simulink model "c00003"  (R2018a)
settings: Solver=ode3  StartTime=0.0  StopTime=10.0  RelTol=1e-3  EnableMultiTasking=on
undefined symbols (not defined in the file): b, DiscIntNeverNeededParam, J, K, L, PosMinimaW3, PosMinimaW4, R
settings Model: Creator=aarrieta  LastModifiedBy=umarkiegi
settings DataIOCC: LimitDataPoints=on  SaveFormat=Array
settings OptimizationCC: LifeSpan=inf
settings DebuggingCC: UnderspecifiedInitializationDetection=Classic  MergeDetectMultiDrivingBlocksExec=none  SolverPrmCheckMsg=warning  StateNameClashWarn=warning  SFUnexpectedBacktrackingDiag=warning  SFNoUnconditionalDefaultTransitionDiag=warning  SFExecutionAtInitializationDiag=none
settings HardwareCC: ProdBitPerPointer=32  ProdBitPerSizeT=32  ProdBitPerPtrDiffT=32  ProdLargestAtomicFloat=None  ProdIntDivRoundTo=Undefined  ProdEndianess=Unspecified  ProdWordSize=32  ProdHWDeviceType=32-bit Generic
settings ModelReferenceCC: PropagateSignalLabelsOutOfModel=off
settings CodeAppCC: StateflowObjectComments=on
settings GRTTargetCC: TargetLangStandard=C89/C90 (ANSI)  GeneratePreprocessorConditionals=Disable all
settings ConfigComp: CovMetricSettings=dw  CovHtmlReporting=on  CovSaveCumulativeToWorkspaceVar=on  CovSaveSingleToWorkspaceVar=on  CovExternalEMLEnable=off  DVMaxTestCaseSteps=20  DVTestSuiteOptimization=CombinedObjectives (Nonlinear Extended)  DVDetectFloatOverflow=off

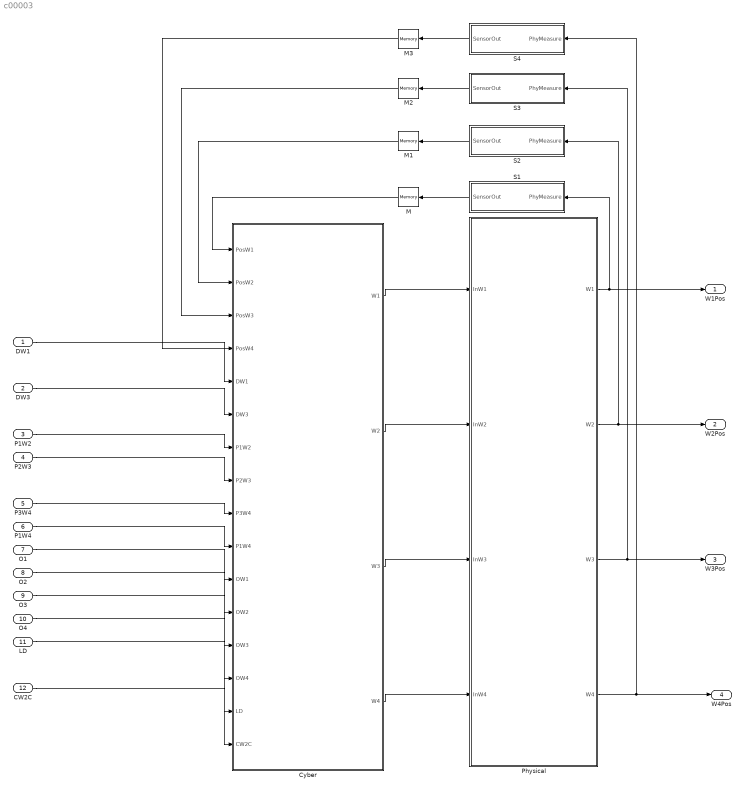
== system c00003 ==
  DW1 : Inport  OutMin=0  OutMax=4  OutDataTypeStr=int8
  DW3 : Inport  Port=2  OutMin=0  OutMax=4  OutDataTypeStr=int8
  P1W2 : Inport  Port=3  OutMin=0  OutMax=4  OutDataTypeStr=int8
  P2W3 : Inport  Port=4  OutMin=0  OutMax=4  OutDataTypeStr=int8
  P3W4 : Inport  Port=5  OutMin=0  OutMax=4  OutDataTypeStr=int8
  P1W4 : Inport  Port=6  OutMin=0  OutMax=4  OutDataTypeStr=int8
  O1 : Inport  Port=7  OutDataTypeStr=boolean
  O2 : Inport  Port=8  OutDataTypeStr=boolean
  O3 : Inport  Port=9  OutDataTypeStr=boolean
  O4 : Inport  Port=10  OutDataTypeStr=boolean
  LD : Inport  Port=11  OutDataTypeStr=boolean
  CW2C : Inport  Port=12  OutMin=0  OutMax=4  OutDataTypeStr=int8
  Cyber : Subsystem
  M{,1..3} (4 alike) : Memory
  Physical : Subsystem
  S1 : Subsystem
  S2 : Subsystem
  S3 : Subsystem
  S4 : Subsystem
  W1Pos : Outport
  W2Pos : Outport  Port=2
  W3Pos : Outport  Port=3
  W4Pos : Outport  Port=4
  wires:
  Cyber/3(W3) -> Physical/3(InW3)
  Physical/1(W1) -> W1Pos/1, S1/1(PhyMeasure)
  Physical/2(W2) -> W2Pos/1, S2/1(PhyMeasure)
  Physical/3(W3) -> W3Pos/1, S3/1(PhyMeasure)
  Physical/4(W4) -> W4Pos/1, S4/1(PhyMeasure)
  M/1 -> Cyber/1(PosW1)
  M1/1 -> Cyber/2(PosW2)
  Cyber/4(W4) -> Physical/4(InW4)
  Cyber/2(W2) -> Physical/2(InW2)
  Cyber/1(W1) -> Physical/1(InW1)
  S4/1(SensorOut) -> M3/1
  M2/1 -> Cyber/3(PosW3)
  S3/1(SensorOut) -> M2/1
  S2/1(SensorOut) -> M1/1
  S1/1(SensorOut) -> M/1
  DW1/1 -> Cyber/5(DW1)
  DW3/1 -> Cyber/6(DW3)
  P1W2/1 -> Cyber/7(P1W2)
  P2W3/1 -> Cyber/8(P2W3)
  P3W4/1 -> Cyber/9(P3W4)
  P1W4/1 -> Cyber/10(P1W4)
  O1/1 -> Cyber/11(OW1)
  O2/1 -> Cyber/12(OW2)
  O3/1 -> Cyber/13(OW3)
  O4/1 -> Cyber/14(OW4)
  LD/1 -> Cyber/15(LD)
  CW2C/1 -> Cyber/16(CW2C)
  M3/1 -> Cyber/4(PosW4)

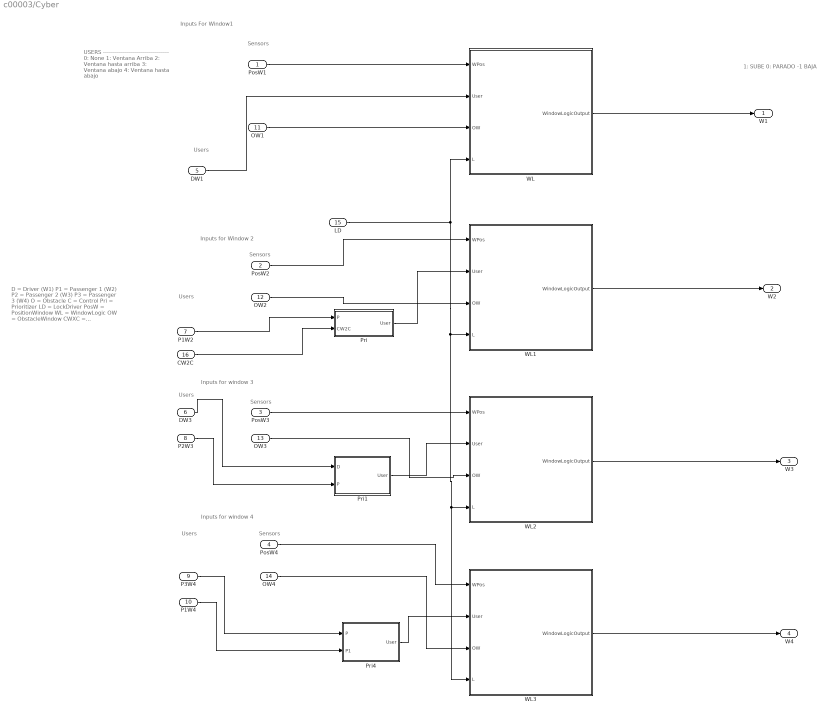
== system c00003/Cyber ==
  note: D = Driver (W1)
      | P1 = Passenger 1 (W2)
      | P2 = Passenger 2 (W3)
      | P3 = Passenger 3 (W4)
      | O = Obstacle
      | C = Control
      | Pri = Prioritizer
      | LD = LockDriver
      | PosW = PositionWindow
      | WL = WindowLogic
      | OW = ObstacleWindow
      | CWXC = ControlWindowXCentralized
      | S = Sensor
      | L = Lock
      | WPos = WindowPosition
      | M = Memory
      | InW = InputWindow
      | WIn = WindowInput
  note: 1: SUBE
      | 0: PARADO
      | -1 BAJA
  note: USERS
      | ---------------------------------
      | 0: None
      | 1: Ventana Arriba
      | 2: Ventana hasta arriba
      | 3: Ventana abajo
      | 4: Ventana hasta abajo
  note: Sensors
  note: Users
  note: Sensors
  note: Users
  note: Sensors
  note: Users
  note: Users
  note: Inputs for window 4
  note: Inputs for window 3
  note: Inputs for Window 2
  note: Inputs For Window1
  note: Sensors
  PosW1 : Inport
  PosW2 : Inport  Port=2
  PosW3 : Inport  Port=3
  PosW4 : Inport  Port=4
  DW1 : Inport  Port=5
  DW3 : Inport  Port=6
  P1W2 : Inport  Port=7
  P2W3 : Inport  Port=8
  P3W4 : Inport  Port=9
  P1W4 : Inport  Port=10
  OW1 : Inport  Port=11
  OW2 : Inport  Port=12
  OW3 : Inport  Port=13
  OW4 : Inport  Port=14
  LD : Inport  Port=15
  CW2C : Inport  Port=16
  Pri : Subsystem
  Pri1 : Subsystem
  Pri4 : Subsystem
  WL : Subsystem
  WL1 : Subsystem
  WL2 : Subsystem
  WL3 : Subsystem
  W1 : Outport
  W2 : Outport  Port=2
  W3 : Outport  Port=3
  W4 : Outport  Port=4
  wires:
  LD/1 -> WL/4(L), WL1/4(L), WL3/4(L), WL2/4(L)
  PosW1/1 -> WL/1(WPos)
  OW1/1 -> WL/3(OW)
  WL/1(WindowLogicOutput) -> W1/1
  Pri/1(User) -> WL1/2(User)
  P1W2/1 -> Pri/1(P)
  PosW2/1 -> WL1/1(WPos)
  OW2/1 -> WL1/3(OW)
  WL1/1(WindowLogicOutput) -> W2/1
  Pri1/1(User) -> WL2/2(User)
  PosW3/1 -> WL2/1(WPos)
  OW3/1 -> WL2/3(OW)
  DW3/1 -> Pri1/1(D)
  P2W3/1 -> Pri1/2(P)
  P3W4/1 -> Pri4/1(P)
  P1W4/1 -> Pri4/2(P1)
  PosW4/1 -> WL3/1(WPos)
  OW4/1 -> WL3/3(OW)
  Pri4/1(User) -> WL3/2(User)
  WL2/1(WindowLogicOutput) -> W3/1
  WL3/1(WindowLogicOutput) -> W4/1
  CW2C/1 -> Pri/2(CW2C)
  DW1/1 -> WL/2(User)

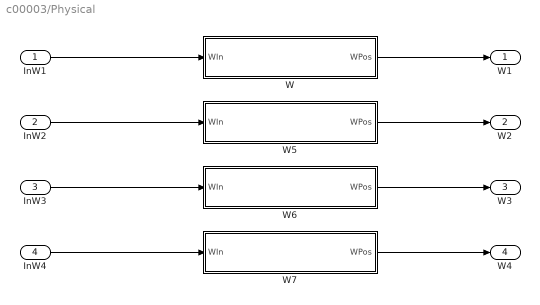
== system c00003/Physical ==
  InW1 : Inport
  InW2 : Inport  Port=2
  InW3 : Inport  Port=3
  InW4 : Inport  Port=4
  W : Subsystem
  W5 : Subsystem
  W6 : Subsystem
  W7 : Subsystem
  W1 : Outport
  W2 : Outport  Port=2
  W3 : Outport  Port=3
  W4 : Outport  Port=4
  wires:
  InW1/1 -> W/1(WIn)
  InW2/1 -> W5/1(WIn)
  InW3/1 -> W6/1(WIn)
  InW4/1 -> W7/1(WIn)
  W/1(WPos) -> W1/1
  W5/1(WPos) -> W2/1
  W6/1(WPos) -> W3/1
  W7/1(WPos) -> W4/1

== system c00003/S1 ==
  PhyMeasure : Inport
  SensorOut : Outport
  wires:
  PhyMeasure/1 -> SensorOut/1

== system c00003/S2 ==
  PhyMeasure : Inport
  SensorOut : Outport
  wires:
  PhyMeasure/1 -> SensorOut/1

== system c00003/S3 ==
  PhyMeasure : Inport
  SensorOut : Outport
  wires:
  PhyMeasure/1 -> SensorOut/1

== system c00003/S4 ==
  PhyMeasure : Inport
  SensorOut : Outport
  wires:
  PhyMeasure/1 -> SensorOut/1

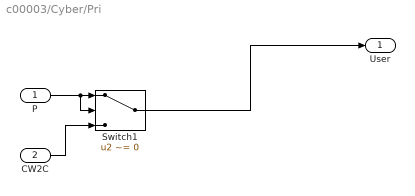
== system c00003/Cyber/Pri ==
  P : Inport
  CW2C : Inport  Port=2
  Switch1 : Switch  Criteria=u2 ~= 0
  User : Outport
  wires:
  P/1 -> Switch1/2, Switch1/1
  CW2C/1 -> Switch1/3
  Switch1/1 -> User/1

== system c00003/Cyber/Pri1 ==
  D : Inport
  P : Inport  Port=2
  Switch : Switch  Criteria=u2 ~= 0
  User : Outport
  wires:
  Switch/1 -> User/1
  D/1 -> Switch/1, Switch/2
  P/1 -> Switch/3

== system c00003/Cyber/Pri4 ==
  P : Inport
  P1 : Inport  Port=2
  Switch1 : Switch  Criteria=u2 ~= 0
  User : Outport
  wires:
  P/1 -> Switch1/2, Switch1/1
  P1/1 -> Switch1/3
  Switch1/1 -> User/1

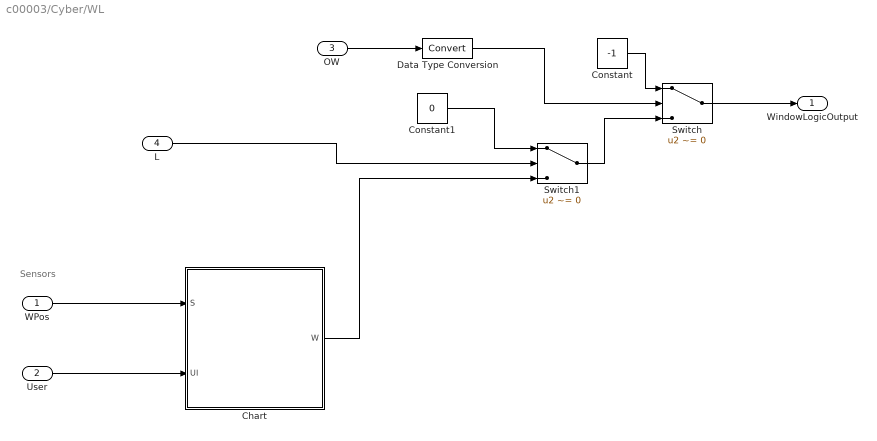
== system c00003/Cyber/WL ==
  note: Sensors
  WPos : Inport
  User : Inport  Port=2
  OW : Inport  Port=3
  L : Inport  Port=4
  Chart : Stateflow chart  TreatAsAtomicUnit=on
  Constant : Constant  Value=-1
  Constant1 : Constant  Value=0
  Data Type Conversion : DataTypeConversion
  Switch : Switch  Criteria=u2 ~= 0  Threshold=1  ZeroCross=off
  Switch1 : Switch  Criteria=u2 ~= 0
  WindowLogicOutput : Outport
  wires:
  OW/1 -> Data Type Conversion/1
  Switch/1 -> WindowLogicOutput/1
  Constant1/1 -> Switch1/1
  Switch1/1 -> Switch/3
  WPos/1 -> Chart/1(S)
  User/1 -> Chart/2(UI)
  Chart/1(W) -> Switch1/3
  Constant/1 -> Switch/1
  Data Type Conversion/1 -> Switch/2
  L/1 -> Switch1/2

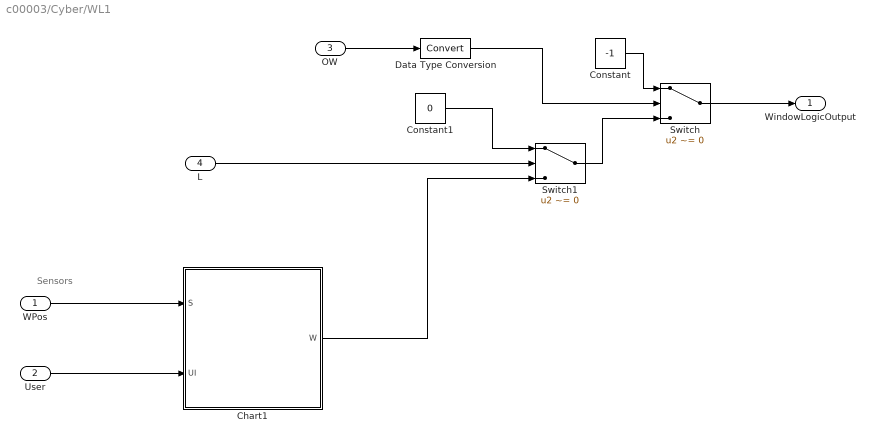
== system c00003/Cyber/WL1 ==
  note: Sensors
  WPos : Inport
  User : Inport  Port=2
  OW : Inport  Port=3
  L : Inport  Port=4
  Chart1 : Stateflow chart  TreatAsAtomicUnit=on
  Constant : Constant  Value=-1
  Constant1 : Constant  Value=0
  Data Type Conversion : DataTypeConversion
  Switch : Switch  Criteria=u2 ~= 0  Threshold=1  ZeroCross=off
  Switch1 : Switch  Criteria=u2 ~= 0
  WindowLogicOutput : Outport
  wires:
  L/1 -> Switch1/2
  Data Type Conversion/1 -> Switch/2
  Constant/1 -> Switch/1
  Chart1/1(W) -> Switch1/3
  User/1 -> Chart1/2(UI)
  WPos/1 -> Chart1/1(S)
  Switch1/1 -> Switch/3
  Constant1/1 -> Switch1/1
  Switch/1 -> WindowLogicOutput/1
  OW/1 -> Data Type Conversion/1

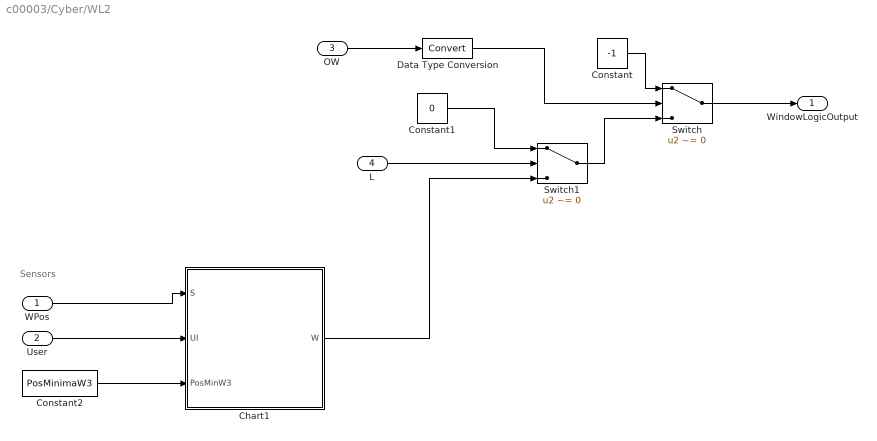
== system c00003/Cyber/WL2 ==
  note: Sensors
  WPos : Inport
  User : Inport  Port=2
  OW : Inport  Port=3
  L : Inport  Port=4
  Chart1 : Stateflow chart  TreatAsAtomicUnit=on
  Constant : Constant  Value=-1
  Constant1 : Constant  Value=0
  Constant2 : Constant  Value=PosMinimaW3
  Data Type Conversion : DataTypeConversion
  Switch : Switch  Criteria=u2 ~= 0  Threshold=1  ZeroCross=off
  Switch1 : Switch  Criteria=u2 ~= 0
  WindowLogicOutput : Outport
  wires:
  OW/1 -> Data Type Conversion/1
  Switch/1 -> WindowLogicOutput/1
  Constant1/1 -> Switch1/1
  Switch1/1 -> Switch/3
  WPos/1 -> Chart1/1(S)
  User/1 -> Chart1/2(UI)
  Chart1/1(W) -> Switch1/3
  Constant/1 -> Switch/1
  Data Type Conversion/1 -> Switch/2
  L/1 -> Switch1/2
  Constant2/1 -> Chart1/3(PosMinW3)

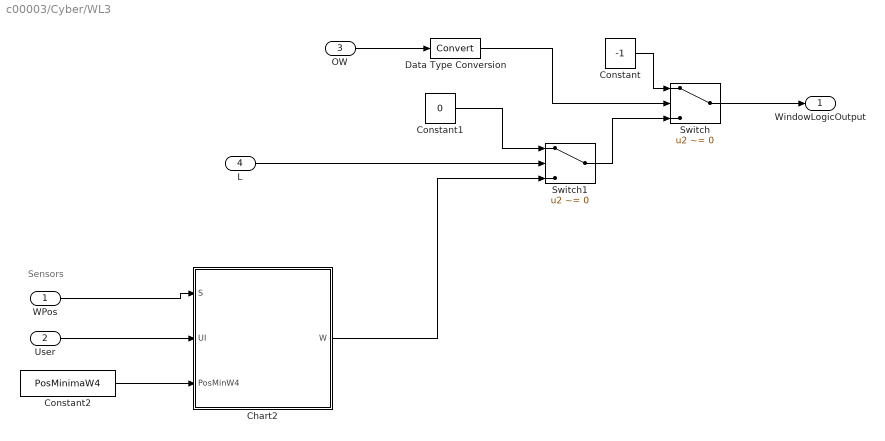
== system c00003/Cyber/WL3 ==
  note: Sensors
  WPos : Inport
  User : Inport  Port=2
  OW : Inport  Port=3
  L : Inport  Port=4
  Chart2 : Stateflow chart  TreatAsAtomicUnit=on
  Constant : Constant  Value=-1
  Constant1 : Constant  Value=0
  Constant2 : Constant  Value=PosMinimaW4
  Data Type Conversion : DataTypeConversion
  Switch : Switch  Criteria=u2 ~= 0  Threshold=1  ZeroCross=off
  Switch1 : Switch  Criteria=u2 ~= 0
  WindowLogicOutput : Outport
  wires:
  L/1 -> Switch1/2
  Data Type Conversion/1 -> Switch/2
  Constant/1 -> Switch/1
  Chart2/1(W) -> Switch1/3
  User/1 -> Chart2/2(UI)
  WPos/1 -> Chart2/1(S)
  Switch1/1 -> Switch/3
  Constant1/1 -> Switch1/1
  Switch/1 -> WindowLogicOutput/1
  OW/1 -> Data Type Conversion/1
  Constant2/1 -> Chart2/3(PosMinW4)

== system c00003/Physical/W ==
  WIn : Inport
  DC_Engine : Subsystem
  Discrete-Time Integrator : DiscreteIntegrator  InitialCondition=5  SampleTime=-1  LimitOutput=on  UpperSaturationLimit=5  LowerSaturationLimit=0  ICPrevOutput=DiscIntNeverNeededParam  ICPrevScaledInput=DiscIntNeverNeededParam
  WPos : Outport
  wires:
  Discrete-Time Integrator/1 -> WPos/1
  DC_Engine/1(Speed) -> Discrete-Time Integrator/1
  WIn/1 -> DC_Engine/1(input)

== system c00003/Physical/W5 ==
  WIn : Inport
  DC_Engine : Subsystem
  Discrete-Time Integrator : DiscreteIntegrator  InitialCondition=5  SampleTime=-1  LimitOutput=on  UpperSaturationLimit=5  LowerSaturationLimit=0  ICPrevOutput=DiscIntNeverNeededParam  ICPrevScaledInput=DiscIntNeverNeededParam
  WPos : Outport
  wires:
  WIn/1 -> DC_Engine/1(input)
  DC_Engine/1(Speed) -> Discrete-Time Integrator/1
  Discrete-Time Integrator/1 -> WPos/1

== system c00003/Physical/W6 ==
  WIn : Inport
  DC_Engine : Subsystem
  Discrete-Time Integrator : DiscreteIntegrator  InitialCondition=5  SampleTime=-1  LimitOutput=on  UpperSaturationLimit=5  LowerSaturationLimit=PosMinimaW3  ICPrevOutput=DiscIntNeverNeededParam  ICPrevScaledInput=DiscIntNeverNeededParam
  WPos : Outport
  wires:
  Discrete-Time Integrator/1 -> WPos/1
  DC_Engine/1(Speed) -> Discrete-Time Integrator/1
  WIn/1 -> DC_Engine/1(input)

== system c00003/Physical/W7 ==
  WIn : Inport
  DC_Engine : Subsystem
  Discrete-Time Integrator : DiscreteIntegrator  InitialCondition=5  SampleTime=-1  LimitOutput=on  UpperSaturationLimit=5  LowerSaturationLimit=PosMinimaW4  ICPrevOutput=DiscIntNeverNeededParam  ICPrevScaledInput=DiscIntNeverNeededParam
  WPos : Outport
  wires:
  WIn/1 -> DC_Engine/1(input)
  DC_Engine/1(Speed) -> Discrete-Time Integrator/1
  Discrete-Time Integrator/1 -> WPos/1

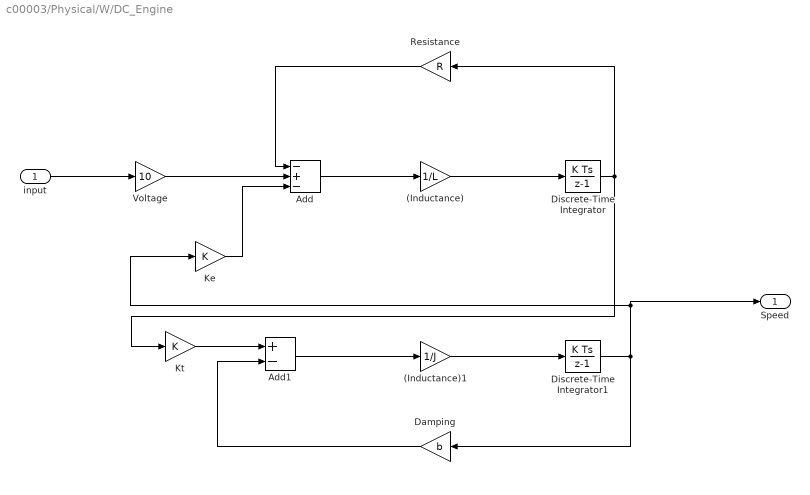
== system c00003/Physical/W/DC_Engine ==
  input : Inport
  (Inductance) : Gain  Gain=1/L
  (Inductance)1 : Gain  Gain=1/J
  Add : Sum  Inputs=-+-
  Add1 : Sum  Inputs=+-
  Damping : Gain  Gain=b
  Discrete-Time Integrator : DiscreteIntegrator  SampleTime=-1  ICPrevOutput=DiscIntNeverNeededParam  ICPrevScaledInput=DiscIntNeverNeededParam
  Discrete-Time Integrator1 : DiscreteIntegrator  SampleTime=-1  ICPrevOutput=DiscIntNeverNeededParam  ICPrevScaledInput=DiscIntNeverNeededParam
  Ke : Gain  Gain=K
  Kt : Gain  Gain=K
  Resistance : Gain  Gain=R
  Voltage : Gain  Gain=10
  Speed : Outport
  wires:
  input/1 -> Voltage/1
  Voltage/1 -> Add/2
  Add/1 -> (Inductance)/1
  Discrete-Time Integrator/1 -> Kt/1, Resistance/1
  Resistance/1 -> Add/1
  Ke/1 -> Add/3
  Kt/1 -> Add1/1
  Add1/1 -> (Inductance)1/1
  (Inductance)1/1 -> Discrete-Time Integrator1/1
  Discrete-Time Integrator1/1 -> Ke/1, Speed/1, Damping/1
  Damping/1 -> Add1/2
  (Inductance)/1 -> Discrete-Time Integrator/1

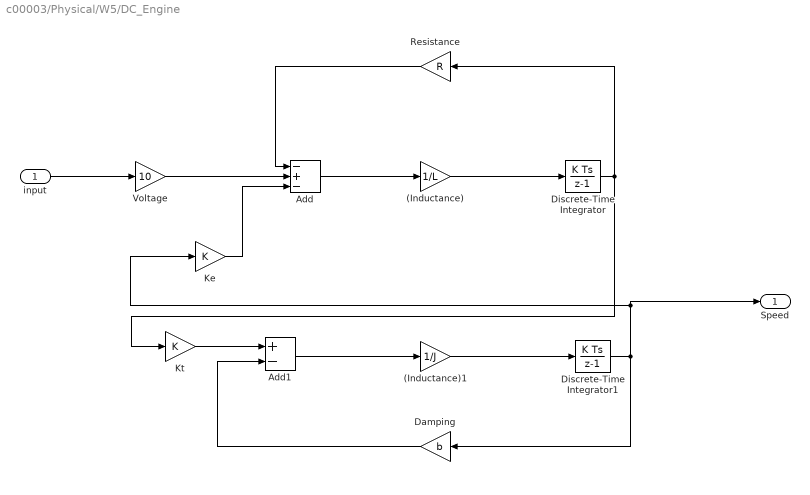
== system c00003/Physical/W5/DC_Engine ==
  input : Inport
  (Inductance) : Gain  Gain=1/L
  (Inductance)1 : Gain  Gain=1/J
  Add : Sum  Inputs=-+-
  Add1 : Sum  Inputs=+-
  Damping : Gain  Gain=b
  Discrete-Time Integrator : DiscreteIntegrator  SampleTime=-1  ICPrevOutput=DiscIntNeverNeededParam  ICPrevScaledInput=DiscIntNeverNeededParam
  Discrete-Time Integrator1 : DiscreteIntegrator  SampleTime=-1  ICPrevOutput=DiscIntNeverNeededParam  ICPrevScaledInput=DiscIntNeverNeededParam
  Ke : Gain  Gain=K
  Kt : Gain  Gain=K
  Resistance : Gain  Gain=R
  Voltage : Gain  Gain=10
  Speed : Outport
  wires:
  Damping/1 -> Add1/2
  Discrete-Time Integrator1/1 -> Damping/1, Speed/1, Ke/1
  (Inductance)1/1 -> Discrete-Time Integrator1/1
  Add1/1 -> (Inductance)1/1
  Kt/1 -> Add1/1
  Ke/1 -> Add/3
  Resistance/1 -> Add/1
  Discrete-Time Integrator/1 -> Resistance/1, Kt/1
  (Inductance)/1 -> Discrete-Time Integrator/1
  Add/1 -> (Inductance)/1
  Voltage/1 -> Add/2
  input/1 -> Voltage/1

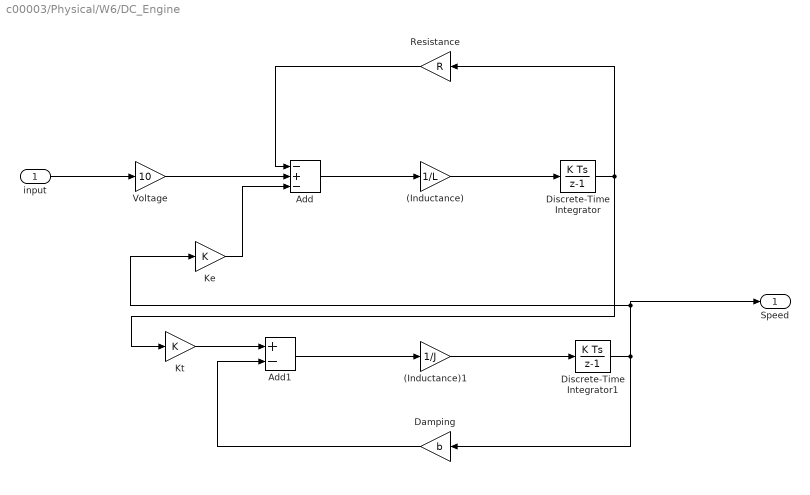
== system c00003/Physical/W6/DC_Engine ==
  input : Inport
  (Inductance) : Gain  Gain=1/L
  (Inductance)1 : Gain  Gain=1/J
  Add : Sum  Inputs=-+-
  Add1 : Sum  Inputs=+-
  Damping : Gain  Gain=b
  Discrete-Time Integrator : DiscreteIntegrator  SampleTime=-1  ICPrevOutput=DiscIntNeverNeededParam  ICPrevScaledInput=DiscIntNeverNeededParam
  Discrete-Time Integrator1 : DiscreteIntegrator  SampleTime=-1  ICPrevOutput=DiscIntNeverNeededParam  ICPrevScaledInput=DiscIntNeverNeededParam
  Ke : Gain  Gain=K
  Kt : Gain  Gain=K
  Resistance : Gain  Gain=R
  Voltage : Gain  Gain=10
  Speed : Outport
  wires:
  input/1 -> Voltage/1
  Voltage/1 -> Add/2
  Add/1 -> (Inductance)/1
  (Inductance)/1 -> Discrete-Time Integrator/1
  Discrete-Time Integrator/1 -> Kt/1, Resistance/1
  Resistance/1 -> Add/1
  Ke/1 -> Add/3
  Kt/1 -> Add1/1
  Add1/1 -> (Inductance)1/1
  (Inductance)1/1 -> Discrete-Time Integrator1/1
  Discrete-Time Integrator1/1 -> Ke/1, Speed/1, Damping/1
  Damping/1 -> Add1/2

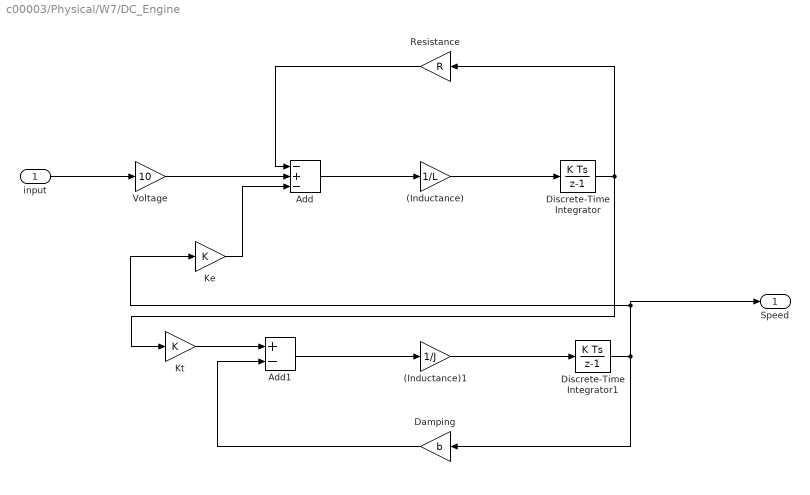
== system c00003/Physical/W7/DC_Engine ==
  input : Inport
  (Inductance) : Gain  Gain=1/L
  (Inductance)1 : Gain  Gain=1/J
  Add : Sum  Inputs=-+-
  Add1 : Sum  Inputs=+-
  Damping : Gain  Gain=b
  Discrete-Time Integrator : DiscreteIntegrator  SampleTime=-1  ICPrevOutput=DiscIntNeverNeededParam  ICPrevScaledInput=DiscIntNeverNeededParam
  Discrete-Time Integrator1 : DiscreteIntegrator  SampleTime=-1  ICPrevOutput=DiscIntNeverNeededParam  ICPrevScaledInput=DiscIntNeverNeededParam
  Ke : Gain  Gain=K
  Kt : Gain  Gain=K
  Resistance : Gain  Gain=R
  Voltage : Gain  Gain=10
  Speed : Outport
  wires:
  Damping/1 -> Add1/2
  Discrete-Time Integrator1/1 -> Damping/1, Speed/1, Ke/1
  (Inductance)1/1 -> Discrete-Time Integrator1/1
  Add1/1 -> (Inductance)1/1
  Kt/1 -> Add1/1
  Ke/1 -> Add/3
  Resistance/1 -> Add/1
  Discrete-Time Integrator/1 -> Resistance/1, Kt/1
  (Inductance)/1 -> Discrete-Time Integrator/1
  Add/1 -> (Inductance)/1
  Voltage/1 -> Add/2
  input/1 -> Voltage/1

== stateflow chart c00003/Cyber/WL/Chart ==
  state Bajand_hasta_abajo
    entry: W = -1;
  state Bajando
    entry: W = -1;
  state Idle
    entry:W = 0;
  state Subiendo_hasta_arriba
    entry: W = 1;
  state Subiendo
    entry: W = 1;
  Subiendo -> Bajand_hasta_abajo [order 4] : [UI==4]
  Bajand_hasta_abajo -> Bajando [order 2] : [UI==3]
  Subiendo -> Bajando [order 3] : [UI==3]
  Bajando -> Bajand_hasta_abajo [order 2] : [UI==4]
  Idle -> Bajando [order 3] : [UI==3&&S>0]
  Subiendo_hasta_arriba -> Bajand_hasta_abajo [order 3] : [UI==4]
  Idle -> Bajand_hasta_abajo [order 4] : [UI==4&&S>0]
  Bajando -> Subiendo [order 3] : [UI==1]
  Subiendo_hasta_arriba -> Bajando [order 4] : [UI==3]
  Bajand_hasta_abajo -> Subiendo [order 4] : [UI==1]
  Bajand_hasta_abajo -> Idle [order 1] : [S<=0]
  Bajand_hasta_abajo -> Subiendo_hasta_arriba [order 3] : [UI==2]
  Bajando -> Idle [order 1] : [S<=0||UI==0]
  Bajando -> Subiendo_hasta_arriba [order 4] : [UI==2]
  (default) -> Idle
  Idle -> Subiendo_hasta_arriba [order 2] : [UI==2&&S<5]
  Idle -> Subiendo [order 1] : [UI == 1&&S<5]
  Subiendo -> Idle [order 1] : [S>=5||UI==0]
  Subiendo_hasta_arriba -> Idle [order 1] : [S >=5]
  Subiendo_hasta_arriba -> Subiendo [order 2] : [UI ==1]
  Subiendo -> Subiendo_hasta_arriba [order 2] : [UI==2]
  data: S input; UI input; W output double

== stateflow chart c00003/Cyber/WL2/Chart1 ==
  state Bajand_hasta_abajo
    entry: W = -1;
  state Bajando
    entry: W = -1;
  state Idle
    entry:W = 0;
  state Subiendo_hasta_arriba
    entry: W = 1;
  state Subiendo
    entry: W = 1;
  Subiendo -> Bajand_hasta_abajo [order 4] : [UI==4]
  Bajand_hasta_abajo -> Bajando [order 2] : [UI==3]
  Subiendo -> Bajando [order 3] : [UI==3]
  Bajando -> Bajand_hasta_abajo [order 2] : [UI==4]
  Idle -> Bajando [order 3] : [UI==3&&S>PosMinW3]
  Subiendo_hasta_arriba -> Bajand_hasta_abajo [order 3] : [UI==4]
  Idle -> Bajand_hasta_abajo [order 4] : [UI==4&&S>PosMinW3]
  Bajando -> Subiendo [order 3] : [UI==1]
  Subiendo_hasta_arriba -> Bajando [order 4] : [UI==3]
  Bajand_hasta_abajo -> Subiendo [order 4] : [UI==1]
  Bajand_hasta_abajo -> Idle [order 1] : [S<=PosMinW3]
  Bajand_hasta_abajo -> Subiendo_hasta_arriba [order 3] : [UI==2]
  Bajando -> Idle [order 1] : [S<=PosMinW3||UI==0]
  Bajando -> Subiendo_hasta_arriba [order 4] : [UI==2]
  (default) -> Idle
  Idle -> Subiendo_hasta_arriba [order 2] : [UI==2&&S<5]
  Idle -> Subiendo [order 1] : [UI == 1&&S<5]
  Subiendo -> Idle [order 1] : [S>=5||UI==0]
  Subiendo_hasta_arriba -> Idle [order 1] : [S >=5]
  Subiendo_hasta_arriba -> Subiendo [order 2] : [UI ==1]
  Subiendo -> Subiendo_hasta_arriba [order 2] : [UI==2]
  data: S input; UI input; W output double; PosMinW3 input

== stateflow chart c00003/Cyber/WL1/Chart1 ==
  state Bajand_hasta_abajo
    entry: W = -1;
  state Bajando
    entry: W = -1;
  state Idle
    entry:W = 0;
  state Subiendo_hasta_arriba
    entry: W = 1;
  state Subiendo
    entry: W = 1;
  Subiendo -> Bajand_hasta_abajo [order 4] : [UI==4]
  Bajand_hasta_abajo -> Bajando [order 2] : [UI==3]
  Subiendo -> Bajando [order 3] : [UI==3]
  Bajando -> Bajand_hasta_abajo [order 2] : [UI==4]
  Idle -> Bajando [order 3] : [UI==3&&S>0]
  Subiendo_hasta_arriba -> Bajand_hasta_abajo [order 3] : [UI==4]
  Idle -> Bajand_hasta_abajo [order 4] : [UI==4&&S>0]
  Bajando -> Subiendo [order 3] : [UI==1]
  Subiendo_hasta_arriba -> Bajando [order 4] : [UI==3]
  Bajand_hasta_abajo -> Subiendo [order 4] : [UI==1]
  Bajand_hasta_abajo -> Idle [order 1] : [S<=0]
  Bajand_hasta_abajo -> Subiendo_hasta_arriba [order 3] : [UI==2]
  Bajando -> Idle [order 1] : [S<=0||UI==0]
  Bajando -> Subiendo_hasta_arriba [order 4] : [UI==2]
  (default) -> Idle
  Idle -> Subiendo_hasta_arriba [order 2] : [UI==2&&S<5]
  Idle -> Subiendo [order 1] : [UI == 1&&S<5]
  Subiendo -> Idle [order 1] : [S>=5||UI==0]
  Subiendo_hasta_arriba -> Idle [order 1] : [S >=5]
  Subiendo_hasta_arriba -> Subiendo [order 2] : [UI ==1]
  Subiendo -> Subiendo_hasta_arriba [order 2] : [UI==2]
  data: S input; UI input; W output double

== stateflow chart c00003/Cyber/WL3/Chart2 ==
  state Bajand_hasta_abajo
    entry: W = -1;
  state Bajando
    entry: W = -1;
  state Idle
    entry:W = 0;
  state Subiendo_hasta_arriba
    entry: W = 1;
  state Subiendo
    entry: W = 1;
  Subiendo -> Bajand_hasta_abajo [order 4] : [UI==4]
  Bajand_hasta_abajo -> Bajando [order 2] : [UI==3]
  Subiendo -> Bajando [order 3] : [UI==3]
  Bajando -> Bajand_hasta_abajo [order 2] : [UI==4]
  Idle -> Bajando [order 3] : [UI==3&&S>PosMinW4]
  Subiendo_hasta_arriba -> Bajand_hasta_abajo [order 3] : [UI==4]
  Idle -> Bajand_hasta_abajo [order 4] : [UI==4&&S>PosMinW4]
  Bajando -> Subiendo [order 3] : [UI==1]
  Subiendo_hasta_arriba -> Bajando [order 4] : [UI==3]
  Bajand_hasta_abajo -> Subiendo [order 4] : [UI==1]
  Bajand_hasta_abajo -> Idle [order 1] : [S<=PosMinW4]
  Bajand_hasta_abajo -> Subiendo_hasta_arriba [order 3] : [UI==2]
  Bajando -> Idle [order 1] : [S<=PosMinW4||UI==0]
  Bajando -> Subiendo_hasta_arriba [order 4] : [UI==2]
  (default) -> Idle
  Idle -> Subiendo_hasta_arriba [order 2] : [UI==2&&S<5]
  Idle -> Subiendo [order 1] : [UI == 1&&S<5]
  Subiendo -> Idle [order 1] : [S>=5||UI==0]
  Subiendo_hasta_arriba -> Idle [order 1] : [S >=5]
  Subiendo_hasta_arriba -> Subiendo [order 2] : [UI ==1]
  Subiendo -> Subiendo_hasta_arriba [order 2] : [UI==2]
  data: S input; UI input; W output double; PosMinW4 input
